simulink model "Task2"  (R2013b)
settings: Solver=ode45  StartTime=0.0  StopTime=1  RelTol=1e-3
settings Model: Creator=barnetdavi  LastModifiedBy=barnetdavi

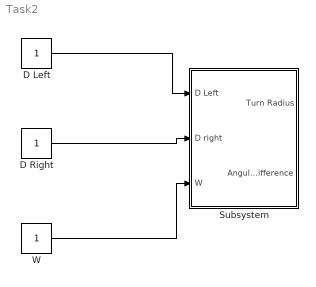
== system Task2 ==
  D Left : Constant
  D Right : Constant
  Subsystem : Subsystem
  W : Constant
  wires:
  D Left/1 -> Subsystem/1(D Left)
  D Right/1 -> Subsystem/2(D right)
  W/1 -> Subsystem/3(W)

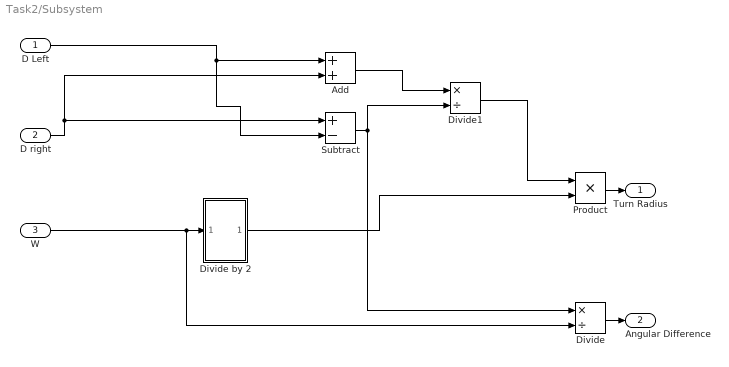
== system Task2/Subsystem ==
  D Left : Inport
  D right : Inport  Port=2
  W : Inport  Port=3
  Add : Sum
  Divide : Product  Inputs=*/
  Divide by 2 : Subsystem
  Divide1 : Product  Inputs=*/
  Product : Product
  Subtract : Sum  Inputs=+-
  Turn Radius : Outport
  Angular Difference : Outport  Port=2
  wires:
  Subtract/1 -> Divide/1, Divide1/2
  Divide by 2/1(Out1) -> Product/2
  Product/1 -> Turn Radius/1
  Divide/1 -> Angular Difference/1
  D right/1 -> Subtract/1, Add/2
  D Left/1 -> Subtract/2, Add/1
  Add/1 -> Divide1/1
  Divide1/1 -> Product/1
  W/1 -> Divide/2, Divide by 2/1(In1)

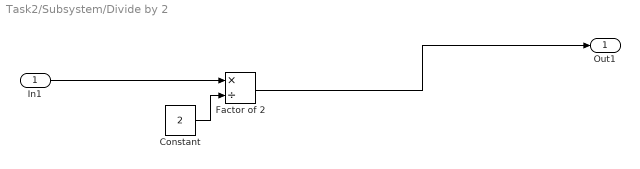
== system Task2/Subsystem/Divide by 2 ==
  In1 : Inport
  Constant : Constant  Value=2
  Factor of 2 : Product  Inputs=*/
  Out1 : Outport
  wires:
  Constant/1 -> Factor of 2/2
  In1/1 -> Factor of 2/1
  Factor of 2/1 -> Out1/1
